simulink model "chap7_10"  (Simulink 3.00)
settings: Solver=ode45  StartTime=0.0  StopTime=10  RelTol=1e-3
undefined symbols (not defined in the file or in its folder): chap7_10f

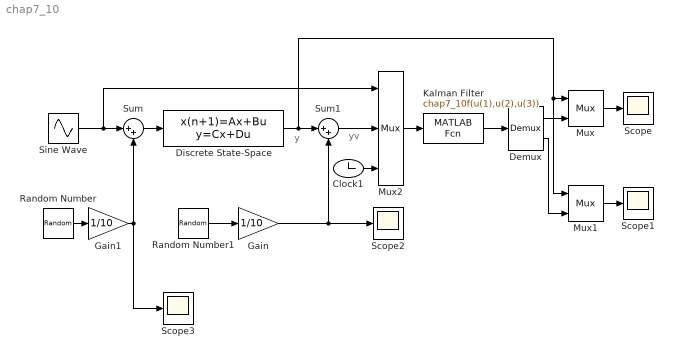
== system chap7_10 ==
  note: y
  note: yv
  Clock1 : Clock
  Demux : Demux  Outputs=2
  Discrete State-Space : DiscreteStateSpace  A=[1.0000 0.0010;0 0.9753]  B=[0.0001;0.1314]  C=[1 0]  D=0  X0=0  SampleTime=0.001
  Gain : Gain  Gain=1/10  SaturateOnIntegerOverflow=on
  Gain1 : Gain  Gain=1/10  SaturateOnIntegerOverflow=on
  Kalman Filter : MATLABFcn  MATLABFcn=chap7_10f(u(1),u(2),u(3))  OutputWidth=2  OutputSignalType=auto
  Mux : Mux  Inputs=2
      settings: DisplayOption=none
  Mux1 : Mux  Inputs=2
      settings: DisplayOption=none
  Mux2 : Mux  Inputs=3
      settings: DisplayOption=none
  Random Number : RandomNumber  Mean=0  Variance=1  Seed=0  SampleTime=0.001
  Random Number1 : RandomNumber  Mean=0  Variance=1  Seed=0  SampleTime=0.001
  Scope{,1..3} (4 alike) : Scope
      Scope settings: TimeRange=1  YMin=-0.5  YMax=3.5  SaveToWorkspace=off  SaveName=ScopeData
      Scope1 settings: TimeRange=1  YMin=0.75  YMax=2.5  SaveToWorkspace=off  SaveName=ScopeData
      Scope2 settings: TimeRange=1  YMin=-3  YMax=3.5  SaveToWorkspace=off  SaveName=ScopeData
      Scope3 settings: TimeRange=1  YMin=-3  YMax=2  SaveToWorkspace=off  SaveName=ScopeData
  Sine Wave : Sin  Amplitude=1  Frequency=1*pi  Phase=0  SampleTime=0.001
  Sum : Sum  Inputs=|++  SaturateOnIntegerOverflow=on
  Sum1 : Sum  Inputs=|++  SaturateOnIntegerOverflow=on
  wires:
  Mux2/1 -> Kalman Filter/1
  Clock1/1 -> Mux2/3
  Sine Wave/1 -> Mux2/1, Sum/1
  Sum/1 -> Discrete State-Space/1
  Sum1/1 -> Mux2/2
  Discrete State-Space/1 -> Sum1/1, Mux/1, Mux1/1
  Random Number/1 -> Gain1/1
  Kalman Filter/1 -> Demux/1
  Gain1/1 -> Sum/2, Scope3/1
  Random Number1/1 -> Gain/1
  Gain/1 -> Sum1/2, Scope2/1
  Demux/2 -> Mux1/2
  Demux/1 -> Mux/2
  Mux/1 -> Scope/1
  Mux1/1 -> Scope1/1
